simulink subsystem "Encoder_SubSystem"  (R2020b)
settings: Solver=VariableStepAuto  StartTime=0.0  StopTime=10.0  RelTol=1e-3
values from neighbouring files (symbols this model uses):
  Ts = T2    (= 0.01)    [PIDAntiWindupDigital.m]    (also in PIDDigital.m = 0.001; StateSpaceControllerNominalCont.m = 0.001; StateSpaceControllerNominalDigital.m = 0.001; StateSpaceControllerNominalDirectDigital.m = 0.05)
undefined symbols (not defined in the file or in its folder): sens
settings Model: Creator=umberto  LastModifiedBy=umbe

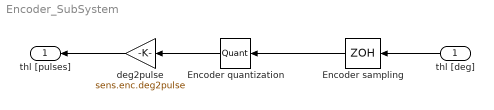
== system Encoder_SubSystem ==
  thl [deg] : Inport
  Encoder quantization : Quantizer  QuantizationInterval=360/sens.enc.ppr
  Encoder sampling : ZeroOrderHold  SampleTime=Ts
  deg2pulse : Gain  Gain=sens.enc.deg2pulse
  thl [pulses] : Outport
  wires:
  Encoder sampling/1 -> Encoder quantization/1
  Encoder quantization/1 -> deg2pulse/1
  deg2pulse/1 -> thl [pulses]/1
  thl [deg]/1 -> Encoder sampling/1
